simulink model "simsystem"  (Simulink 5.0)
settings: Solver=ode45  StartTime=0.0  StopTime=10.0  RelTol=1e-3
values from neighbouring files (symbols this model uses):
  a = l*l-(j/(mc+mp))    (= -0.0106644567937)    [init_para.m]
  dzcv = 0.0079311    [init_para.m]
  fc = 0.9    [init_para.m]
  fp = 0.000107443    [init_para.m]
  fs = 2.28133    [init_para.m]
  g = 9.81    [init_para.m]
  j = 0.0135735    [init_para.m]
  l = 0.0167903    [init_para.m]
  mi = (mc+mp)*l    (= 0.020819972)    [init_para.m]
  xc = 2.5    [init_para.m]
  yc = 2.5    [init_para.m]
settings Model: LastModifiedBy=AD

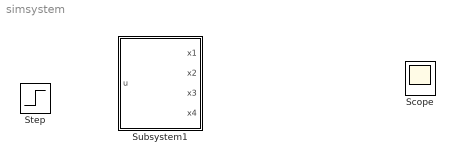
== system simsystem ==
  Scope : Scope
      settings: TimeRange=10  YMin=-100  YMax=500
  Step : Step  SampleTime=0
  Subsystem1 : Subsystem

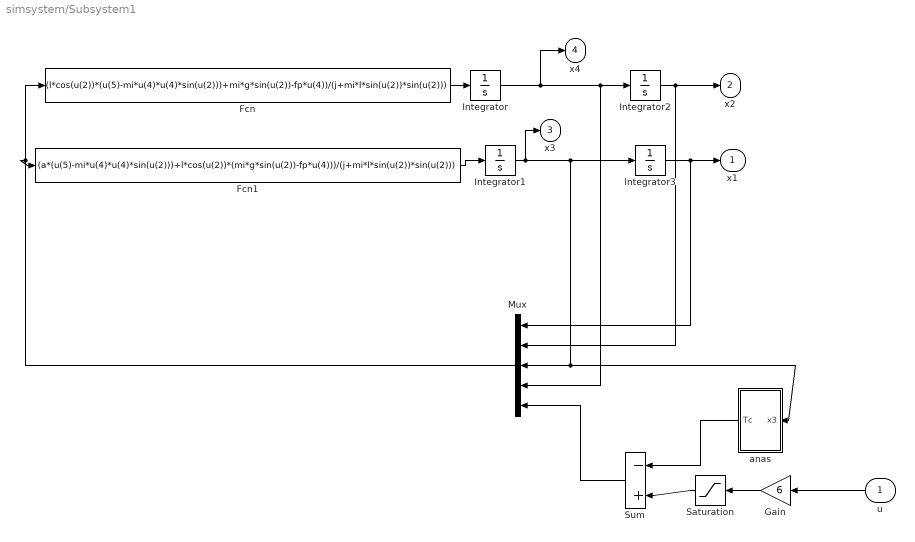
== system simsystem/Subsystem1 ==
  u : Inport  Orientation=left
  Fcn : Fcn  Expr=(l*cos(u(2))*(u(5)-mi*u(4)*u(4)*sin(u(2)))+mi*g*sin(u(2))-fp*u(4))/(j+mi*l*sin(u(2))*sin(u(2)))
  Fcn1 : Fcn  Expr=(a*(u(5)-mi*u(4)*u(4)*sin(u(2)))+l*cos(u(2))*(mi*g*sin(u(2))-fp*u(4)))/(j+mi*l*sin(u(2))*sin(u(2)))
  Gain : Gain  Orientation=left  Gain=6  SaturateOnIntegerOverflow=on
  Integrator{,1..3} (4 alike) : Integrator
  Mux : Mux  Orientation=left  Inputs=5
  Saturation : Saturate  Orientation=left  UpperLimit=17  LowerLimit=-17
  Sum : Sum  Orientation=left  Inputs=|-+  SaturateOnIntegerOverflow=on
  anas : Subsystem  Orientation=left
  x1 : Outport
  x2 : Outport  Port=2
  x3 : Outport  Port=3
  x4 : Outport  Port=4
  wires:
  Fcn/1 -> Integrator/1
  Fcn1/1 -> Integrator1/1
  Integrator/1 -> Integrator2/1, Mux/4, x4/1
  Integrator1/1 -> Integrator3/1, Mux/3, anas/1(x3), x3/1
  Integrator2/1 -> x2/1, Mux/2
  Integrator3/1 -> x1/1, Mux/1
  Mux/1 -> Fcn1/1, Fcn/1
  Sum/1 -> Mux/5
  Gain/1 -> Saturation/1
  Saturation/1 -> Sum/2
  u/1 -> Gain/1
  anas/1(Tc) -> Sum/1

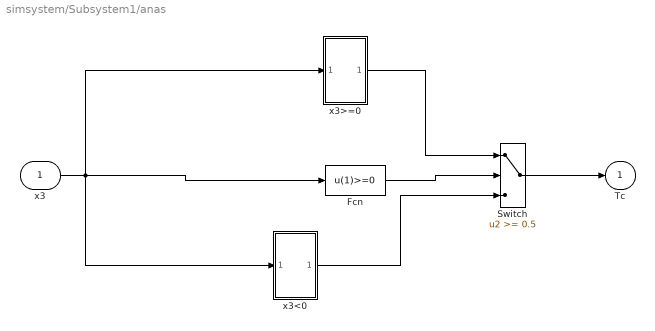
== system simsystem/Subsystem1/anas ==
  x3 : Inport
  Fcn : Fcn  Expr=u(1)>=0
  Switch : Switch  Threshold=0.5  SaturateOnIntegerOverflow=on
  x3<0 : Subsystem
  x3>=0 : Subsystem
  Tc : Outport
  wires:
  Switch/1 -> Tc/1
  Fcn/1 -> Switch/2
  x3/1 -> Fcn/1, x3>=0/1(In1), x3<0/1(In1)
  x3>=0/1(out1) -> Switch/1
  x3<0/1(out1) -> Switch/3

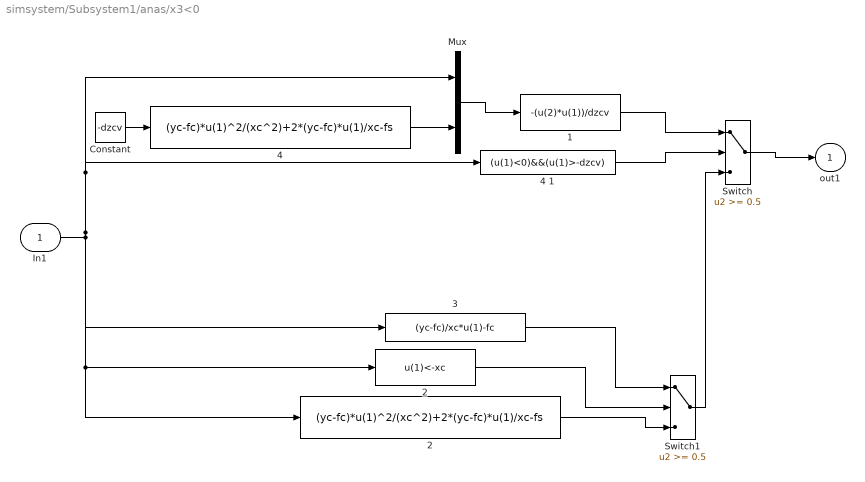
== system simsystem/Subsystem1/anas/x3<0 ==
  In1 : Inport
  1 : Fcn  Expr=-(u(2)*u(1))/dzcv
  2 : Fcn  Expr=u(1)<-xc
  "2 " : Fcn  Expr=(yc-fc)*u(1)^2/(xc^2)+2*(yc-fc)*u(1)/xc-fs
  3 : Fcn  Expr=(yc-fc)/xc*u(1)-fc
  "4 " : Fcn  Expr=(yc-fc)*u(1)^2/(xc^2)+2*(yc-fc)*u(1)/xc-fs
  4 1 : Fcn  Expr=(u(1)<0)&&(u(1)>-dzcv)
  Constant : Constant  Value=-dzcv
  Mux : Mux  Inputs=2
  Switch : Switch  Threshold=0.5  SaturateOnIntegerOverflow=on
  Switch1 : Switch  Threshold=0.5  SaturateOnIntegerOverflow=on
  out1 : Outport
  wires:
  1/1 -> Switch/1
  3/1 -> Switch1/1
  2/1 -> Switch1/2
  "2 "/1 -> Switch1/3
  Switch1/1 -> Switch/3
  Mux/1 -> 1/1
  "4 "/1 -> Mux/2
  In1/1 -> 3/1, 2/1, "2 "/1, Mux/1, 4 1/1
  Constant/1 -> "4 "/1
  4 1/1 -> Switch/2
  Switch/1 -> out1/1

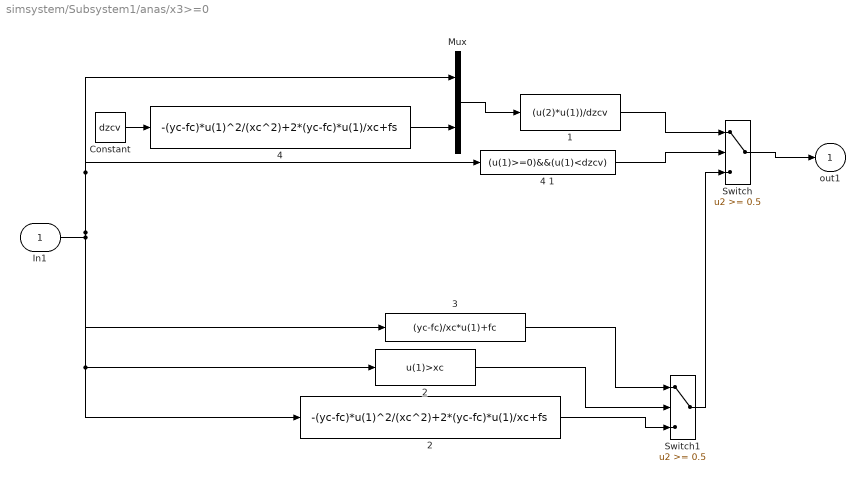
== system simsystem/Subsystem1/anas/x3>=0 ==
  In1 : Inport
  1 : Fcn  Expr=(u(2)*u(1))/dzcv
  2 : Fcn  Expr=u(1)>xc
  "2 " : Fcn  Expr=-(yc-fc)*u(1)^2/(xc^2)+2*(yc-fc)*u(1)/xc+fs
  3 : Fcn  Expr=(yc-fc)/xc*u(1)+fc
  "4 " : Fcn  Expr=-(yc-fc)*u(1)^2/(xc^2)+2*(yc-fc)*u(1)/xc+fs
  4 1 : Fcn  Expr=(u(1)>=0)&&(u(1)<dzcv)
  Constant : Constant  Value=dzcv
  Mux : Mux  Inputs=2
  Switch : Switch  Threshold=0.5  SaturateOnIntegerOverflow=on
  Switch1 : Switch  Threshold=0.5  SaturateOnIntegerOverflow=on
  out1 : Outport
  wires:
  1/1 -> Switch/1
  3/1 -> Switch1/1
  2/1 -> Switch1/2
  "2 "/1 -> Switch1/3
  Switch1/1 -> Switch/3
  Mux/1 -> 1/1
  "4 "/1 -> Mux/2
  In1/1 -> 3/1, 2/1, "2 "/1, Mux/1, 4 1/1
  Constant/1 -> "4 "/1
  4 1/1 -> Switch/2
  Switch/1 -> out1/1
